simulink model "Kinematic_Bicycle_Model"  (R2021a)
settings: Solver=VariableStepAuto  StartTime=0.0  StopTime=30  RelTol=1e-3
model workspace (MAT data in the model file):
  radius = 8
libraries: simulink x1
settings Model: Creator=AK  LastModifiedBy=AK

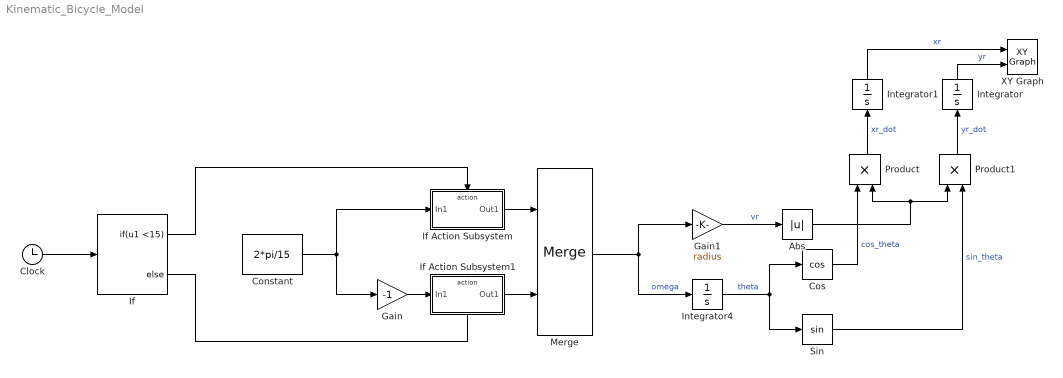
== system Kinematic_Bicycle_Model ==
  Abs : Abs
  Clock : Clock
  Constant : Constant  Value=2*pi/15
  Cos : Trigonometry  Operator=cos
  Gain : Gain  Gain=-1
  Gain1 : Gain  Gain=radius
  If : If  IfExpression=u1 <15
  If Action Subsystem : Subsystem  TreatAsAtomicUnit=on
  If Action Subsystem1 : Subsystem  TreatAsAtomicUnit=on
  Integrator : Integrator
  Integrator1 : Integrator
  Integrator4 : Integrator  InitialCondition=pi/2
  Merge : Merge
  Product : Product
  Product1 : Product
  Sin : Trigonometry
  XY Graph : simulink/Sinks/XY Graph  xmin=-20  xmax=20  ymin=-20  ymax=20  st=-1
  wires:
  Product/1 -> Integrator1/1  "xr_dot"
  Merge/1 -> Gain1/1, Integrator4/1  "omega"
  Integrator4/1 -> Cos/1, Sin/1  "theta"
  Cos/1 -> Product/1  "cos_theta"
  Sin/1 -> Product1/2  "sin_theta"
  Product1/1 -> Integrator/1  "yr_dot"
  Constant/1 -> If Action Subsystem/1(In1), Gain/1
  Clock/1 -> If/1
  If/1 -> If Action Subsystem/Action
  Gain/1 -> If Action Subsystem1/1(In1)
  Integrator/1 -> XY Graph/2  "yr"
  Integrator1/1 -> XY Graph/1  "xr"
  If/2 -> If Action Subsystem1/Action
  If Action Subsystem1/1(Out1) -> Merge/2
  If Action Subsystem/1(Out1) -> Merge/1
  Gain1/1 -> Abs/1  "vr"
  Abs/1 -> Product/2, Product1/1

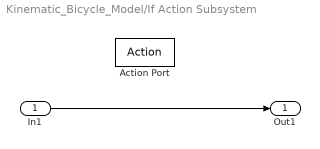
== system Kinematic_Bicycle_Model/If Action Subsystem ==
  In1 : Inport
  Action Port : ActionPort  ActionPortLabel=if(u1 <15)
  Out1 : Outport
  wires:
  In1/1 -> Out1/1

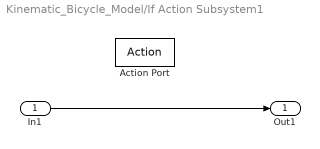
== system Kinematic_Bicycle_Model/If Action Subsystem1 ==
  In1 : Inport
  Action Port : ActionPort  ActionPortLabel=else
  Out1 : Outport
  wires:
  In1/1 -> Out1/1
